simulink model "Ejer10_RespuestaEscalonUnitario"  (R2023b)
settings: Solver=VariableStepAuto  StartTime=0  StopTime=50  RelTol=1e-3
settings Model: Creator=alfre  LastModifiedBy=alfre

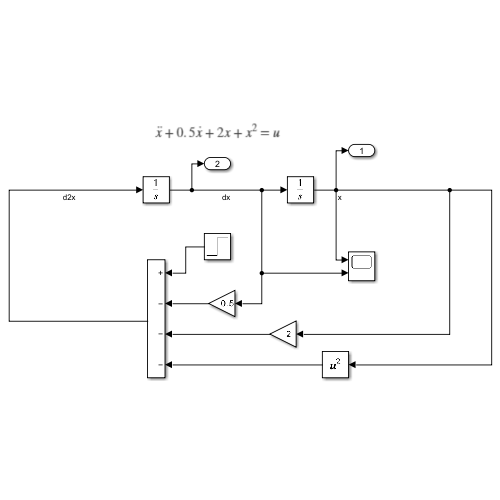
[thumbnail: Simulink's stored preview of the top-level diagram]
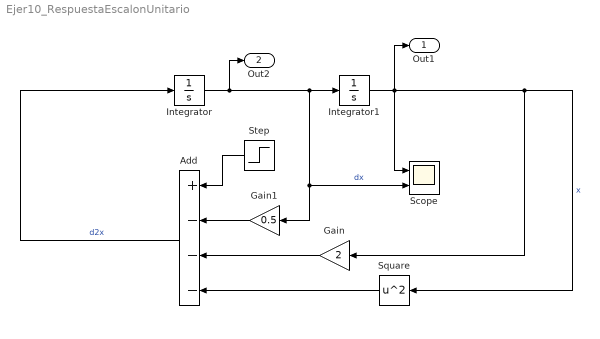
== system Ejer10_RespuestaEscalonUnitario ==
  Add : Sum  Inputs=+---
  Gain : Gain  Gain=2
  Gain1 : Gain  Gain=0.5
  Integrator : Integrator
  Integrator1 : Integrator
  Scope : Scope  NumInputPorts=2
  Square : Math  Operator=square
  Step : Step  SampleTime=0
  Out1 : Outport
  Out2 : Outport  Port=2
  wires:
  Add/1 -> Integrator/1  "d2x"
  Integrator/1 -> Out2/1, Gain1/1, Scope/2, Integrator1/1  "dx"
  Integrator1/1 -> Square/1, Gain/1, Scope/1, Out1/1  "x"
  Square/1 -> Add/4
  Gain/1 -> Add/3
  Gain1/1 -> Add/2
  Step/1 -> Add/1
